simulink model "gm_spec_avg_CRD_vs2"  (R2025b)
settings: Solver=FixedStepDiscrete  StartTime=0.0  StopTime=0.0005  FixedStep=1.66666666666667e-08  RelTol=1e-3
undefined symbols (not defined in the file or in its folder): chirp_counts, chirp_outputs, clk, clk_enable, FFT_LENGTH, Fs, h, reset, specAvg
libraries: simulink x30, hdlmdlgenlib x4, dsphdlsigops2 x2, dsphdlxfrm2 x1, hdlsllib x1, vivadosimlib x1
(part 1 of 2)
settings Model: FPTRunName=BaselineRun  Creator=caleb  LastModifiedBy=caleb
settings OptimizationCC: BlockReduction=off  ConditionallyExecuteInputs=off  DefaultParameterBehavior=Inlined  OptimizeBlockIOStorage=off  EnhancedBackFolding=on  PassReuseOutputArgsThreshold=0.0  OptimizeBlockOrder=speed  DifferentSizesBufferReuse=on
settings DebuggingCC: SignalRangeChecking=warning  AlgebraicLoopMsg=error  InheritedTsInSrcMsg=none  SingleTaskRateTransMsg=error  ParameterTunabilityLossMsg=error
settings HardwareCC: ProdBitPerPointer=32.0  ProdBitPerSizeT=32.0  ProdBitPerPtrDiffT=32.0  ProdLargestAtomicFloat=None  ProdIntDivRoundTo=Undefined  ProdEndianess=Unspecified  ProdWordSize=32.0  ProdHWDeviceType=ASIC/FPGA->ASIC/FPGA  TargetBitPerPointer=64.0  TargetBitPerSizeT=64.0  TargetBitPerPtrDiffT=64.0  TargetLongLongMode=on  TargetIntDivRoundTo=Zero  TargetEndianess=LittleEndian  TargetWordSize=64.0  TargetHWDeviceType=Generic->Custom  ProdEqTarget=off
settings SFSimCC: MATLABDynamicMemAlloc=off
settings RTWCC: GPUComputeCapability=3.5
settings CodeAppCC: ForceParamTrailComments=on  MaxIdLength=256.0  OperatorAnnotations=on

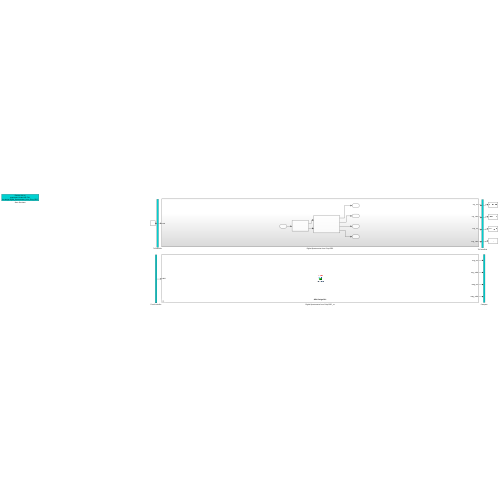
[thumbnail: Simulink's stored preview of the top-level diagram]
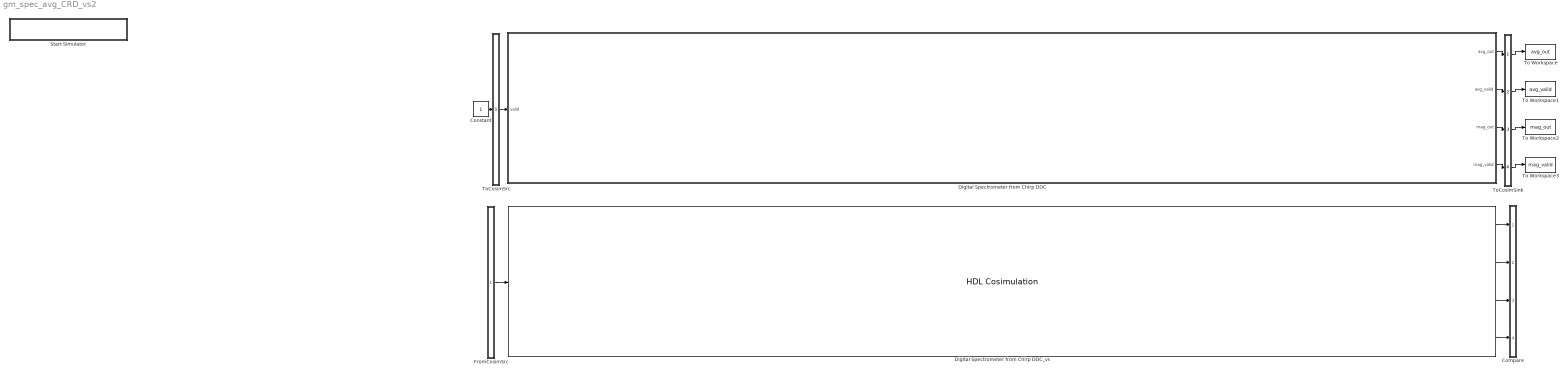
== system gm_spec_avg_CRD_vs2 ==
  Compare : Subsystem
      mask Display: disp('')
  Constant : Constant  OutDataTypeStr=boolean  SampleTime=1/Fs
  Digital Spectrometer from Chirp DDC : Subsystem
  Digital Spectrometer from Chirp DDC_vs : vivadosimlib/HDL Cosimulation  PortPaths=/Digital_Spectrometer_from_Chirp_DDC/valid;/Digital_Spectrometer_from_Chirp_DDC/avg_out;/Digital_Spectrometer_from_Chirp_DDC/avg_valid;/Digital_Spectrometer_from_Chirp_DDC/mag_out;/Digital_Spectrometer_from_Chirp_DDC/mag_valid  PortModes=[1 2 2 2 2 ]  PortTimes=[-1 3.333333333333333403075202767094908917755446964292787015438079834e-08 3.333333333333333403075202767094908917755446964292787015438079834e-08 3.333333333333333403075202767094908917755446964292787015438079834e-08 3.333333333333333403075202767094908917755446964292787015438079834e-08 ]  PortSigns=[-1 1 0 1 0 ]  PortFracLengths=[0,4,0,15,0]  PortWordLengths=[-1,32,1,26,1]  PortHDLWordSizes=[1,32,1,26,1]  CommLocal=on  CommSharedMemory=on  CommPortNumber=4449  CommShowInfo=on  ClockPaths=clk;clk_enable;reset;  ClockModes=[2 4 3]  ClockTimes=[1e-08 3.7e-08 2.7e-08]  TclPostSimCommand="puts \"done\""  TimingMode=ns  TimingScaleFactor=600000000  idxCellArray={'UNUSED_VAR'}  CosimBypass=Full Simulation  AllowDirectFeedthrough=on  ProductName=EDA Simulator Link VS  RunAutoTimescale=off  HdlClocks=0  PreRunTime=40  PreRunTimeUnit=ns
  FromCosimSrc : Subsystem
      mask Display: disp('')
  Start Simulator : Subsystem
      settings: OpenFcn=|
      | cosimDirName = pwd;
      | cd 'C:\VHDL\spec_avg\hdlsrc\spec_avg_CRD';
      | [s,r] = system('vivado -mode batch -source gm_spec_avg_CRD_vs.tcl','-echo');
      | cd (cosimDirName);
      | clear cosimDirName;
      | if s
      |    error('Failed to create Vivado HDL design DLL using script gm_spec_avg_CRD_vs.tcl.');
      | end
      mask Display: disp('Double-click to\nregenerate Vivado HDL DLL\nfor design Digital_Spectrometer_from_Chirp_DDC')
  To Workspace : ToWorkspace  VariableName=avg_out  SampleTime=-1
      settings: Save2DSignal=2-D array (concatenate along first dimension)
  To Workspace1 : ToWorkspace  VariableName=avg_valid  SampleTime=-1
      settings: Save2DSignal=2-D array (concatenate along first dimension)
  To Workspace2 : ToWorkspace  VariableName=mag_out  SampleTime=-1
      settings: Save2DSignal=2-D array (concatenate along first dimension)
  To Workspace3 : ToWorkspace  VariableName=mag_valid  SampleTime=-1
      settings: Save2DSignal=2-D array (concatenate along first dimension)
  ToCosimSink : Subsystem
      mask Display: disp('')
  ToCosimSrc : Subsystem
      mask Display: disp('')
  wires:
  ToCosimSrc/1(out1) -> Digital Spectrometer from Chirp DDC/1(valid)
  Digital Spectrometer from Chirp DDC/1(avg_out) -> ToCosimSink/1(in1)
  Digital Spectrometer from Chirp DDC/2(avg_valid) -> ToCosimSink/2(in2)
  Digital Spectrometer from Chirp DDC/3(mag_out) -> ToCosimSink/3(in3)
  Digital Spectrometer from Chirp DDC/4(mag_valid) -> ToCosimSink/4(in4)
  Constant/1 -> ToCosimSrc/1(in1)
  ToCosimSink/1(out1) -> To Workspace/1
  ToCosimSink/2(out2) -> To Workspace1/1
  ToCosimSink/3(out3) -> To Workspace2/1
  ToCosimSink/4(out4) -> To Workspace3/1
  FromCosimSrc/1(out1) -> Digital Spectrometer from Chirp DDC_vs/1
  Digital Spectrometer from Chirp DDC_vs/1 -> Compare/1(in1)
  Digital Spectrometer from Chirp DDC_vs/2 -> Compare/2(in2)
  Digital Spectrometer from Chirp DDC_vs/3 -> Compare/3(in3)
  Digital Spectrometer from Chirp DDC_vs/4 -> Compare/4(in4)

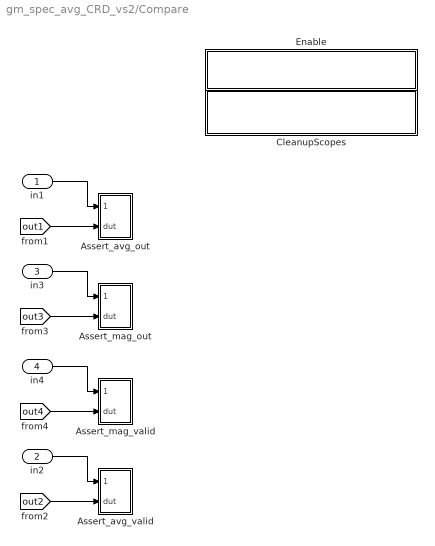
== system gm_spec_avg_CRD_vs2/Compare ==
  in1 : Inport
  in2 : Inport  Port=2
  in3 : Inport  Port=3
  in4 : Inport  Port=4
  Assert_avg_out : Subsystem
  Assert_avg_valid : Subsystem
  Assert_mag_out : Subsystem
  Assert_mag_valid : Subsystem
  CleanupScopes : Subsystem
      settings: OpenFcn=|
      | blkName = gcb; %self block
      | idx = regexp(blkName, '/CleanupScopes$', 'once');
      | blkParent = blkName(1:idx-1);
      | blks=find_system(blkParent, 'LookUnderMasks', 'all','blocktype', 'Scope');
      | for itr = 1:length(blks)
      | 	 hScopeCfg = get_param(blks{itr},'ScopeConfiguration');
      | 	 hScopeCfg.Visible = ~ hScopeCfg.Visible;
      | end
      | drawnow;
      mask Display: fprintf(message('hdlcoder:cosim:vnl_dblclick').getString());
  Enable : Subsystem
      settings: OpenFcn=|
      | blkName = gcb;
      | idx = regexp(blkName, '/Enable$', 'once');
      | blkParent = blkName(1:idx-1);
      | blks=find_system(blkParent, 'LookUnderMasks', 'all','blocktype', 'Assertion');
      | e = get_param(blks{1}, 'Enabled');
      | if strcmp(e, 'on'), f= 'off';, else, f = 'on';, end
      | for ii=1:length(blks), set_param(blks{ii}, 'Enabled', f);, end
      | set_param(gcb, 'MaskDisplay',['fprintf(message(''hdlcoder:cosim:vnl_dblclick_assertions'',','''',upper(e),'''',').getString())']);
      mask Display: fprintf(message('hdlcoder:cosim:vnl_dblclick_assertions','OFF').getString());
  wires:
  in1/1 -> Assert_avg_out/1(cosim)
  [out4] -> Assert_mag_valid/2(dut)
  [out1] -> Assert_avg_out/2(dut)
  in3/1 -> Assert_mag_out/1(cosim)
  [out2] -> Assert_avg_valid/2(dut)
  [out3] -> Assert_mag_out/2(dut)
  in4/1 -> Assert_mag_valid/1(cosim)
  in2/1 -> Assert_avg_valid/1(cosim)

== system gm_spec_avg_CRD_vs2/Digital Spectrometer from Chirp DDC ==
  valid : Inport  OutDataTypeStr=boolean  PortDimensions=1  SampleTime=1.66666666666667e-08
  DDC : Subsystem
  Digital Spectrometer : Subsystem
  avg_out : Outport  SampleTime=3.33333333333333e-08
  avg_valid : Outport  Port=2  SampleTime=3.33333333333333e-08
  mag_out : Outport  Port=3  SampleTime=3.33333333333333e-08
  mag_valid : Outport  Port=4  SampleTime=3.33333333333333e-08
  wires:
  Digital Spectrometer/4(mag_valid) -> mag_valid/1
  Digital Spectrometer/3(mag_out) -> mag_out/1
  Digital Spectrometer/2(avg_valid) -> avg_valid/1
  DDC/2(valid_out) -> Digital Spectrometer/2(valid_in)
  DDC/1(signal_out) -> Digital Spectrometer/1(signal_in)
  valid/1 -> DDC/1(valid)
  Digital Spectrometer/1(avg_out) -> avg_out/1

== system gm_spec_avg_CRD_vs2/FromCosimSrc ==
  out1 : Outport
  wires:
  [in1] -> out1/1

== system gm_spec_avg_CRD_vs2/Start Simulator ==

== system gm_spec_avg_CRD_vs2/ToCosimSink ==
  in1 : Inport
  in2 : Inport  Port=2
  in3 : Inport  Port=3
  in4 : Inport  Port=4
  out1 : Outport
  out2 : Outport  Port=2
  out3 : Outport  Port=3
  out4 : Outport  Port=4
  tag scope: out1=global, out2=global, out3=global, out4=global
  wires:
  in1/1 -> out1/1, [out1]
  in2/1 -> out2/1, [out2]
  in3/1 -> out3/1, [out3]
  in4/1 -> out4/1, [out4]

== system gm_spec_avg_CRD_vs2/ToCosimSrc ==
  in1 : Inport
  out1 : Outport
  tag scope: in1=global
  wires:
  in1/1 -> out1/1, [in1]

== system gm_spec_avg_CRD_vs2/Compare/Assert_avg_out ==
  cosim : Inport
  dut : Inport  Port=2
  AssertEq : Assertion
  Compare To Zero : simulink/Logic and Bit Operations/Compare To Zero  relop===  OutDataTypeStr=boolean
  Relational Operator : RelationalOperator  Operator===  OutDataTypeStr=boolean  InputSameDT=off
  compare: avg_out : Scope  NumInputPorts=3
      settings: ActiveDisplayYMinimum=-29.585937499999993  ActiveDisplayYMaximum=229.3984375
  wires:
  Compare To Zero/1 -> compare: avg_out/3  "err"
  Relational Operator/1 -> Compare To Zero/1, AssertEq/1
  cosim/1 -> compare: avg_out/1, Relational Operator/1  "cosim"
  dut/1 -> compare: avg_out/2, Relational Operator/2  "dut ref"

== system gm_spec_avg_CRD_vs2/Compare/Assert_avg_valid ==
  cosim : Inport
  dut : Inport  Port=2
  AssertEq : Assertion
  Compare To Zero : simulink/Logic and Bit Operations/Compare To Zero  relop===  OutDataTypeStr=boolean
  Relational Operator : RelationalOperator  Operator===  OutDataTypeStr=boolean  InputSameDT=off
  compare: avg_valid : Scope  NumInputPorts=3
      settings: ActiveDisplayYMinimum=-5  ActiveDisplayYMaximum=5
  wires:
  Compare To Zero/1 -> compare: avg_valid/3  "err"
  Relational Operator/1 -> Compare To Zero/1, AssertEq/1
  cosim/1 -> compare: avg_valid/1, Relational Operator/1  "cosim"
  dut/1 -> compare: avg_valid/2, Relational Operator/2  "dut ref"

== system gm_spec_avg_CRD_vs2/Compare/Assert_mag_out ==
  cosim : Inport
  dut : Inport  Port=2
  AssertEq : Assertion
  Compare To Zero : simulink/Logic and Bit Operations/Compare To Zero  relop===  OutDataTypeStr=boolean
  Relational Operator : RelationalOperator  Operator===  OutDataTypeStr=boolean  InputSameDT=off
  compare: mag_out : Scope  NumInputPorts=3
      settings: ActiveDisplayYMinimum=-5  ActiveDisplayYMaximum=5
  wires:
  Compare To Zero/1 -> compare: mag_out/3  "err"
  Relational Operator/1 -> Compare To Zero/1, AssertEq/1
  cosim/1 -> compare: mag_out/1, Relational Operator/1  "cosim"
  dut/1 -> compare: mag_out/2, Relational Operator/2  "dut ref"

== system gm_spec_avg_CRD_vs2/Compare/Assert_mag_valid ==
  cosim : Inport
  dut : Inport  Port=2
  AssertEq : Assertion
  Compare To Zero : simulink/Logic and Bit Operations/Compare To Zero  relop===  OutDataTypeStr=boolean
  Relational Operator : RelationalOperator  Operator===  OutDataTypeStr=boolean  InputSameDT=off
  compare: mag_valid : Scope  NumInputPorts=3
      settings: ActiveDisplayYMinimum=-5  ActiveDisplayYMaximum=5
  wires:
  Compare To Zero/1 -> compare: mag_valid/3  "err"
  Relational Operator/1 -> Compare To Zero/1, AssertEq/1
  cosim/1 -> compare: mag_valid/1, Relational Operator/1  "cosim"
  dut/1 -> compare: mag_valid/2, Relational Operator/2  "dut ref"

== system gm_spec_avg_CRD_vs2/Compare/CleanupScopes ==

== system gm_spec_avg_CRD_vs2/Compare/Enable ==

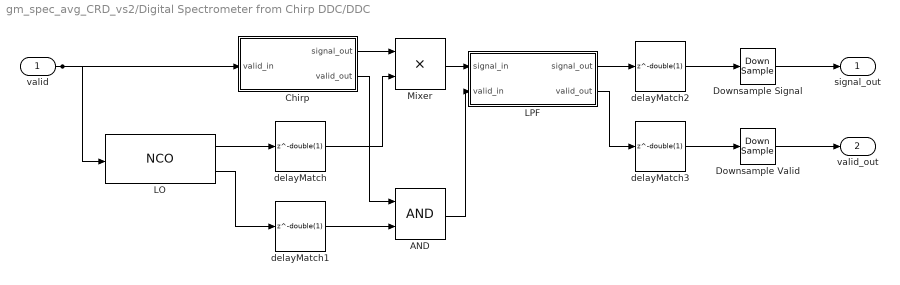
== system gm_spec_avg_CRD_vs2/Digital Spectrometer from Chirp DDC/DDC ==
  valid : Inport  OutDataTypeStr=boolean  PortDimensions=1  SampleTime=1.66666666666667e-08
  AND : Logic  AllPortsSameDT=off  OutDataTypeStr=boolean  SampleTime=1.66666666666667e-08
  Chirp : Subsystem
  Downsample Signal : DownSample  N=double(2)  phase=double(0)  RateOptions=Allow multirate processing  AllowArbitraryFixedInput=on
  Downsample Valid : DownSample  N=double(2)  phase=double(0)  RateOptions=Allow multirate processing  AllowArbitraryFixedInput=on
  LO : dsphdlsigops2/NCO  PhaseIncrementSource=Property  PhaseIncrement=phIncr  PhaseOffsetSource=Property  PhaseOffset=phOff  DitherSource=Property  NumDitherBits=ditherBits  SamplesPerFrame=1  LUTCompress=off  ResetAction=off  Waveform=Cosine  PhasePort=off  SimulateUsing=Code generation  AccumulatorWL=N  PhaseQuantization=on  NumQuantizerAccumulatorBits=Q  OutputDataType=Binary point scaling  OutputWL=16  OutputFL=14
  LPF : Subsystem
  Mixer : Product  Inputs=**  OutDataTypeStr=fixdt(1, 16, 14)  SampleTime=1.66666666666667e-08
  delayMatch{,1..3} (4 alike) : Delay  DelayLength=double(1)  InitialCondition=0  SampleTime=1.66666666666667e-08
  signal_out : Outport  SampleTime=3.33333333333333e-08  VectorParamsAs1DForOutWhenUnconnected=off
  valid_out : Outport  Port=2  SampleTime=3.33333333333333e-08  VectorParamsAs1DForOutWhenUnconnected=off
  wires:
  Downsample Valid/1 -> valid_out/1
  Downsample Signal/1 -> signal_out/1
  delayMatch3/1 -> Downsample Valid/1
  delayMatch2/1 -> Downsample Signal/1
  LPF/2(valid_out) -> delayMatch3/1
  LPF/1(signal_out) -> delayMatch2/1
  AND/1 -> LPF/2(valid_in)
  Mixer/1 -> LPF/1(signal_in)
  delayMatch1/1 -> AND/2
  Chirp/2(valid_out) -> AND/1
  Chirp/1(signal_out) -> Mixer/1
  LO/2 -> delayMatch1/1
  LO/1 -> delayMatch/1
  delayMatch/1 -> Mixer/2
  valid/1 -> LO/1, Chirp/1(valid_in)

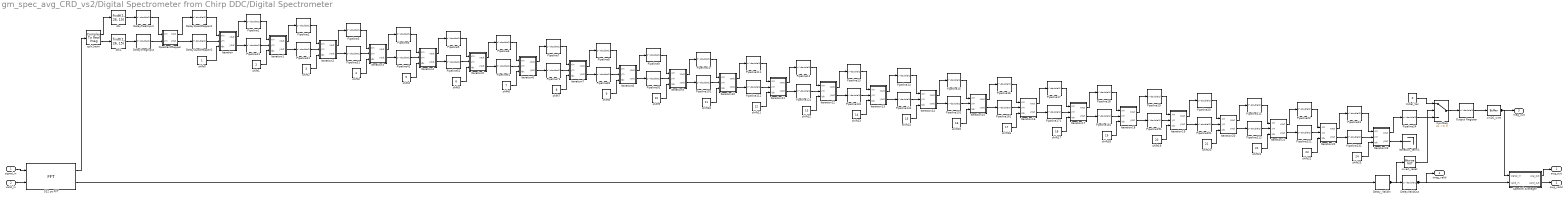
== system gm_spec_avg_CRD_vs2/Digital Spectrometer from Chirp DDC/Digital Spectrometer ==
  signal_in : Inport  OutDataTypeStr=fixdt(1, 16, 15)  PortDimensions=1  SampleTime=3.33333333333333e-08
  valid_in : Inport  Port=2  OutDataTypeStr=boolean  PortDimensions=1  SampleTime=3.33333333333333e-08
  512 pt FFT : dsphdlxfrm2/FFT  Architecture=Streaming Radix 2^2  FFTLengthSource=Property  FFTLength=FFT_LENGTH  FFTLengthMax=1024  ComplexMultiplication=Use 4 multipliers and 2 adders  BitReversedOutput=off  BitReversedInput=off  Normalize=off  SimulateUsing=Code generation  RoundingMethod=Floor  ResetInputPort=off  StartOutputPort=off  EndOutputPort=off
  DelayImagInput : Delay  DelayLength=double(1)  InitialCondition=0  SampleTime=3.33333333333333e-08
  DelayQuadMapper1 : Delay  DelayLength=double(1)  InitialCondition=0  SampleTime=3.33333333333333e-08
  DelayQuadMapper2 : Delay  DelayLength=double(1)  InitialCondition=0  SampleTime=3.33333333333333e-08
  DelayRealInput : Delay  DelayLength=double(1)  InitialCondition=0  SampleTime=3.33333333333333e-08
  DelayValidOut : Delay  DelayLength=double(1)  InitialCondition=0  SampleTime=3.33333333333333e-08
  Delay_ValidIn : Delay  DelayLength=double(27)  InitialCondition=0  SampleTime=3.33333333333333e-08
  Initial_Val : Constant  Value=0  OutDataTypeStr=fixdt(1, 26, 15)  SampleTime=3.33333333333333e-08
  Iteration : Subsystem
  Iteration1 : Subsystem
  Iteration10 : Subsystem
  Iteration11 : Subsystem
  Iteration12 : Subsystem
  Iteration13 : Subsystem
  Iteration14 : Subsystem
  Iteration15 : Subsystem
  Iteration16 : Subsystem
  Iteration17 : Subsystem
  Iteration18 : Subsystem
  Iteration19 : Subsystem
  Iteration2 : Subsystem
  Iteration20 : Subsystem
  Iteration21 : Subsystem
  Iteration22 : Subsystem
  Iteration23 : Subsystem
  Iteration3 : Subsystem
  Iteration4 : Subsystem
  Iteration5 : Subsystem
  Iteration6 : Subsystem
  Iteration7 : Subsystem
  Iteration8 : Subsystem
  Iteration9 : Subsystem
  Iteration_term1 : Terminator
  Output Register : Delay  DelayLength=double(1)  InitialCondition=0  SampleTime=3.33333333333333e-08
  Pipeline{1..24,31,41,51,61,71,81,91,101,111..112,121,131,141,151,161,171,181,191,201,211..212,221,231} (47 alike) : Delay  DelayLength=double(1)  InitialCondition=0  SampleTime=3.33333333333333e-08
  QuadrantMapper : Subsystem
  Spectral Averager : Subsystem
  cplx2reim : ComplexToRealImag  SampleTime=3.33333333333333e-08
  dtc : DataTypeConversion  OutDataTypeStr=fixdt(1, 26, 15)  SampleTime=3.33333333333333e-08  SaturateOnIntegerOverflow=off  RndMeth=Floor
  dtc1 : DataTypeConversion  OutDataTypeStr=fixdt(1, 26, 15)  SampleTime=3.33333333333333e-08  SaturateOnIntegerOverflow=off  RndMeth=Floor
  invert_reset : simulink/Logic and Bit Operations/Bitwise Operator  logicop=NOT  UseBitMask=off  BitMask=double(0)  BitMaskRealWorld=Real World Value
  muxMag : Switch  Criteria=u2 ~= 0  Threshold="fi(0,0,1,0,\"hex\",\"0\")"  OutDataTypeStr=fixdt(1, 26, 15)  SampleTime=3.33333333333333e-08  SaturateOnIntegerOverflow=off  InputSameDT=off
  shift0 : Constant  VectorParams1D=off  OutDataTypeStr=fixdt(0, 6, 0)  SampleTime=3.33333333333333e-08
  shift1 : Constant  Value=2  VectorParams1D=off  OutDataTypeStr=fixdt(0, 6, 0)  SampleTime=3.33333333333333e-08
  shift10 : Constant  Value=11  VectorParams1D=off  OutDataTypeStr=fixdt(0, 6, 0)  SampleTime=3.33333333333333e-08
  shift11 : Constant  Value=12  VectorParams1D=off  OutDataTypeStr=fixdt(0, 6, 0)  SampleTime=3.33333333333333e-08
  shift12 : Constant  Value=13  VectorParams1D=off  OutDataTypeStr=fixdt(0, 6, 0)  SampleTime=3.33333333333333e-08
  shift13 : Constant  Value=14  VectorParams1D=off  OutDataTypeStr=fixdt(0, 6, 0)  SampleTime=3.33333333333333e-08
  shift14 : Constant  Value=15  VectorParams1D=off  OutDataTypeStr=fixdt(0, 6, 0)  SampleTime=3.33333333333333e-08
  shift15 : Constant  Value=16  VectorParams1D=off  OutDataTypeStr=fixdt(0, 6, 0)  SampleTime=3.33333333333333e-08
  shift16 : Constant  Value=17  VectorParams1D=off  OutDataTypeStr=fixdt(0, 6, 0)  SampleTime=3.33333333333333e-08
  shift17 : Constant  Value=18  VectorParams1D=off  OutDataTypeStr=fixdt(0, 6, 0)  SampleTime=3.33333333333333e-08
  shift18 : Constant  Value=19  VectorParams1D=off  OutDataTypeStr=fixdt(0, 6, 0)  SampleTime=3.33333333333333e-08
  shift19 : Constant  Value=20  VectorParams1D=off  OutDataTypeStr=fixdt(0, 6, 0)  SampleTime=3.33333333333333e-08
  shift2 : Constant  Value=3  VectorParams1D=off  OutDataTypeStr=fixdt(0, 6, 0)  SampleTime=3.33333333333333e-08
  shift20 : Constant  Value=21  VectorParams1D=off  OutDataTypeStr=fixdt(0, 6, 0)  SampleTime=3.33333333333333e-08
  shift21 : Constant  Value=22  VectorParams1D=off  OutDataTypeStr=fixdt(0, 6, 0)  SampleTime=3.33333333333333e-08
  shift22 : Constant  Value=23  VectorParams1D=off  OutDataTypeStr=fixdt(0, 6, 0)  SampleTime=3.33333333333333e-08
  shift23 : Constant  Value=24  VectorParams1D=off  OutDataTypeStr=fixdt(0, 6, 0)  SampleTime=3.33333333333333e-08
  shift3 : Constant  Value=4  VectorParams1D=off  OutDataTypeStr=fixdt(0, 6, 0)  SampleTime=3.33333333333333e-08
  shift4 : Constant  Value=5  VectorParams1D=off  OutDataTypeStr=fixdt(0, 6, 0)  SampleTime=3.33333333333333e-08
  shift5 : Constant  Value=6  VectorParams1D=off  OutDataTypeStr=fixdt(0, 6, 0)  SampleTime=3.33333333333333e-08
  shift6 : Constant  Value=7  VectorParams1D=off  OutDataTypeStr=fixdt(0, 6, 0)  SampleTime=3.33333333333333e-08
  shift7 : Constant  Value=8  VectorParams1D=off  OutDataTypeStr=fixdt(0, 6, 0)  SampleTime=3.33333333333333e-08
  shift8 : Constant  Value=9  VectorParams1D=off  OutDataTypeStr=fixdt(0, 6, 0)  SampleTime=3.33333333333333e-08
  shift9 : Constant  Value=10  VectorParams1D=off  OutDataTypeStr=fixdt(0, 6, 0)  SampleTime=3.33333333333333e-08
  xin26_wire : hdlmdlgenlib/Buffer
  avg_out : Outport  SampleTime=3.33333333333333e-08
  avg_valid : Outport  Port=2  SampleTime=3.33333333333333e-08
  mag_out : Outport  Port=3  SampleTime=3.33333333333333e-08
  mag_valid : Outport  Port=4  SampleTime=3.33333333333333e-08
  wires:
  Spectral Averager/2(valid_out) -> avg_valid/1
  Spectral Averager/1(avg_out) -> avg_out/1
  xin26_wire/1 -> mag_out/1, Spectral Averager/1(signal_in)
  Output Register/1 -> xin26_wire/1
  muxMag/1 -> Output Register/1
  DelayValidOut/1 -> mag_valid/1, Spectral Averager/2(valid_in)
  Pipeline24/1 -> muxMag/3
  Initial_Val/1 -> muxMag/1
  Delay_ValidIn/1 -> DelayValidOut/1, invert_reset/1
  Iteration23/2(yout) -> Iteration_term1/1
  Iteration23/1(xout) -> Pipeline24/1
  shift23/1 -> Iteration23/3(idx)
  Pipeline231/1 -> Iteration23/2(yin)
  Pipeline23/1 -> Iteration23/1(xin)
  Iteration22/2(yout) -> Pipeline231/1
  Iteration22/1(xout) -> Pipeline23/1
  shift22/1 -> Iteration22/3(idx)
  Pipeline221/1 -> Iteration22/2(yin)
  Pipeline22/1 -> Iteration22/1(xin)
  Iteration21/2(yout) -> Pipeline221/1
  Iteration21/1(xout) -> Pipeline22/1
  shift21/1 -> Iteration21/3(idx)
  Pipeline211/1 -> Iteration21/1(xin)
  Iteration20/2(yout) -> Pipeline212/1
  Iteration20/1(xout) -> Pipeline211/1
  shift20/1 -> Iteration20/3(idx)
  Pipeline20/1 -> Iteration20/1(xin)
  Iteration19/1(xout) -> Pipeline20/1
  shift19/1 -> Iteration19/3(idx)
  Pipeline191/1 -> Iteration19/2(yin)
  Pipeline19/1 -> Iteration19/1(xin)
  Iteration18/1(xout) -> Pipeline19/1
  shift18/1 -> Iteration18/3(idx)
  Pipeline212/1 -> Iteration21/2(yin)
  Pipeline181/1 -> Iteration18/2(yin)
  Pipeline18/1 -> Iteration18/1(xin)
  Iteration17/2(yout) -> Pipeline181/1
  Pipeline17/1 -> Iteration17/1(xin)
  Iteration16/2(yout) -> Pipeline171/1
  Iteration16/1(xout) -> Pipeline17/1
  shift16/1 -> Iteration16/3(idx)
  Pipeline161/1 -> Iteration16/2(yin)
  Pipeline16/1 -> Iteration16/1(xin)
  Iteration15/2(yout) -> Pipeline161/1
  Iteration15/1(xout) -> Pipeline16/1
  shift15/1 -> Iteration15/3(idx)
  Pipeline151/1 -> Iteration15/2(yin)
  Pipeline15/1 -> Iteration15/1(xin)
  Iteration14/2(yout) -> Pipeline151/1
  Iteration14/1(xout) -> Pipeline15/1
  shift14/1 -> Iteration14/3(idx)
  Pipeline141/1 -> Iteration14/2(yin)
  Pipeline14/1 -> Iteration14/1(xin)
  Iteration13/2(yout) -> Pipeline141/1
  shift13/1 -> Iteration13/3(idx)
  Pipeline131/1 -> Iteration13/2(yin)
  Pipeline13/1 -> Iteration13/1(xin)
  Iteration12/2(yout) -> Pipeline131/1
  Iteration12/1(xout) -> Pipeline13/1
  shift12/1 -> Iteration12/3(idx)
  Pipeline12/1 -> Iteration12/1(xin)
  Iteration11/1(xout) -> Pipeline12/1
  shift11/1 -> Iteration11/3(idx)
  Pipeline112/1 -> Iteration11/2(yin)
  Iteration10/2(yout) -> Pipeline112/1
  Iteration10/1(xout) -> Pipeline111/1
  shift10/1 -> Iteration10/3(idx)
  Iteration9/1(xout) -> Pipeline10/1
  Pipeline9/1 -> Iteration9/1(xin)
  Iteration8/2(yout) -> Pipeline91/1
  Pipeline8/1 -> Iteration8/1(xin)
  shift7/1 -> Iteration7/3(idx)
  Pipeline7/1 -> Iteration7/1(xin)
  Pipeline6/1 -> Iteration6/1(xin)
  Iteration7/2(yout) -> Pipeline81/1
  Pipeline101/1 -> Iteration10/2(yin)
  Iteration5/1(xout) -> Pipeline6/1
  shift5/1 -> Iteration5/3(idx)
  Pipeline91/1 -> Iteration9/2(yin)
  Pipeline5/1 -> Iteration5/1(xin)
  shift6/1 -> Iteration6/3(idx)
  Iteration11/2(yout) -> Pipeline121/1
  Pipeline201/1 -> Iteration20/2(yin)
  Iteration6/2(yout) -> Pipeline71/1
  Pipeline41/1 -> Iteration4/2(yin)
  Pipeline4/1 -> Iteration4/1(xin)
  Pipeline171/1 -> Iteration17/2(yin)
  Iteration3/2(yout) -> Pipeline41/1
  invert_reset/1 -> muxMag/2
  Iteration3/1(xout) -> Pipeline4/1
  Pipeline61/1 -> Iteration6/2(yin)
  shift8/1 -> Iteration8/3(idx)
  shift3/1 -> Iteration3/3(idx)
  Pipeline31/1 -> Iteration3/2(yin)
  Iteration18/2(yout) -> Pipeline191/1
  Pipeline3/1 -> Iteration3/1(xin)
  shift4/1 -> Iteration4/3(idx)
  Pipeline71/1 -> Iteration7/2(yin)
  Iteration2/2(yout) -> Pipeline31/1
  Iteration2/1(xout) -> Pipeline3/1
  shift2/1 -> Iteration2/3(idx)
  Pipeline111/1 -> Iteration11/1(xin)
  Pipeline51/1 -> Iteration5/2(yin)
  Iteration1/2(yout) -> Pipeline21/1
  Iteration6/1(xout) -> Pipeline7/1
  Iteration1/1(xout) -> Pipeline2/1
  shift1/1 -> Iteration1/3(idx)
  Iteration17/1(xout) -> Pipeline18/1
  Pipeline10/1 -> Iteration10/1(xin)
  Pipeline11/1 -> Iteration1/2(yin)
  Pipeline1/1 -> Iteration1/1(xin)
  Pipeline21/1 -> Iteration2/2(yin)
  Iteration7/1(xout) -> Pipeline8/1
  Iteration8/1(xout) -> Pipeline9/1
  Iteration/2(yout) -> Pipeline11/1
  Pipeline121/1 -> Iteration12/2(yin)
  Pipeline2/1 -> Iteration2/1(xin)
  Iteration19/2(yout) -> Pipeline201/1
  shift9/1 -> Iteration9/3(idx)
  shift0/1 -> Iteration/3(idx)
  Iteration5/2(yout) -> Pipeline61/1
  DelayQuadMapper2/1 -> Iteration/2(yin)
  Pipeline81/1 -> Iteration8/2(yin)
  DelayQuadMapper1/1 -> Iteration/1(xin)
  Iteration13/1(xout) -> Pipeline14/1
  QuadrantMapper/1(xout) -> DelayQuadMapper1/1
  DelayImagInput/1 -> QuadrantMapper/2(yin)
  DelayRealInput/1 -> QuadrantMapper/1(xin)
  shift17/1 -> Iteration17/3(idx)
  QuadrantMapper/2(yout) -> DelayQuadMapper2/1
  Iteration9/2(yout) -> Pipeline101/1
  dtc1/1 -> DelayImagInput/1
  Iteration4/1(xout) -> Pipeline5/1
  dtc/1 -> DelayRealInput/1
  cplx2reim/1 -> dtc/1
  Iteration4/2(yout) -> Pipeline51/1
  Iteration/1(xout) -> Pipeline1/1
  valid_in/1 -> 512 pt FFT/2
  512 pt FFT/1 -> cplx2reim/1
  512 pt FFT/2 -> Delay_ValidIn/1
  cplx2reim/2 -> dtc1/1
  signal_in/1 -> 512 pt FFT/1

== system gm_spec_avg_CRD_vs2/Digital Spectrometer from Chirp DDC/DDC/Chirp ==
  valid_in : Inport  OutDataTypeStr=boolean  PortDimensions=1  SampleTime=1.66666666666667e-08
  1-D Lookup Table1 : Subsystem
  Constant : Constant  Value=35.791015625  OutDataTypeStr=fixdt(0, 16, 10)  SampleTime=1.66666666666667e-08
  Counter Limited : Subsystem  mask(Counter Limited){uplimit=double(30000), tsamp=double(1.6666666666666667e-08)}
      mask prompts: uplimit "Simulink:masks:UpperLimit_MP"; tsamp "Simulink:masks:SampleTime_MP"
      mask help: Simulink:masks:CounterLimited_MD
      mask init:
      | nbits = double(16);
      | tsamp = double(1.6666666666666667e-08);
      | uplimit = double(30000);
  NCO1 : dsphdlsigops2/NCO  PhaseIncrementSource=Input port  PhaseIncrement=phIncr  PhaseOffsetSource=Property  PhaseOffset=phOff  DitherSource=Property  NumDitherBits=ditherBits  SamplesPerFrame=1  LUTCompress=off  ResetAction=off  Waveform=Cosine  PhasePort=off  SimulateUsing=Code generation  AccumulatorWL=N  PhaseQuantization=on  NumQuantizerAccumulatorBits=Q  OutputDataType=Binary point scaling  OutputWL=16  OutputFL=14
  Product : Product  Inputs=**  OutDataTypeStr=uint32  SampleTime=1.66666666666667e-08
  delayMatch : Delay  DelayLength=double(1)  InitialCondition=0  SampleTime=1.66666666666667e-08
  signal_out : Outport  SampleTime=1.66666666666667e-08
  valid_out : Outport  Port=2  SampleTime=1.66666666666667e-08
  wires:
  NCO1/2 -> valid_out/1
  delayMatch/1 -> NCO1/2
  Product/1 -> NCO1/1
  valid_in/1 -> delayMatch/1
  1-D Lookup Table1/1(Out1) -> Product/2
  Counter Limited/1(y) -> 1-D Lookup Table1/1(In1)
  Constant/1 -> Product/1
  NCO1/1 -> signal_out/1

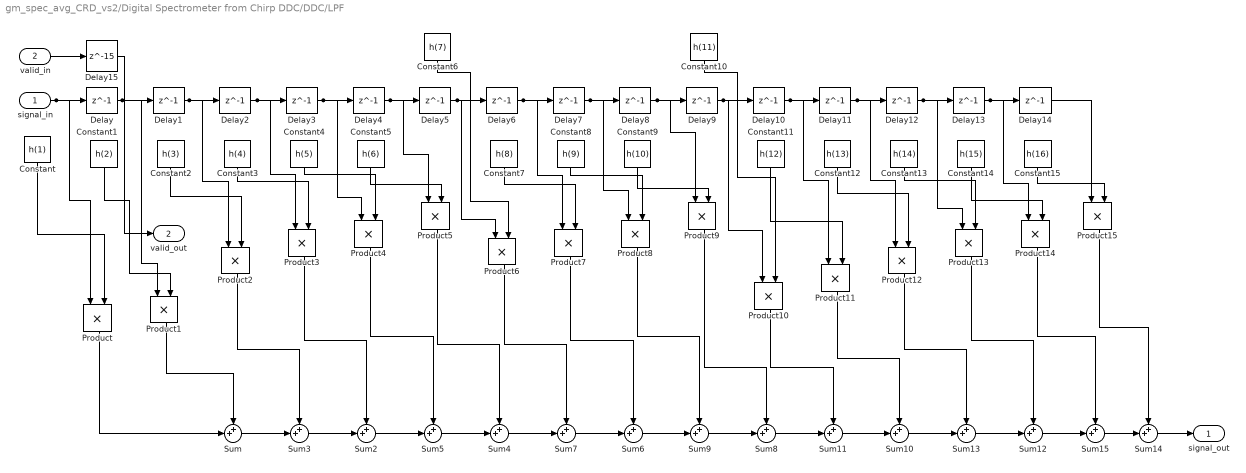
== system gm_spec_avg_CRD_vs2/Digital Spectrometer from Chirp DDC/DDC/LPF ==
  signal_in : Inport  OutDataTypeStr=fixdt(1, 16, 14)  PortDimensions=1  SampleTime=1.66666666666667e-08
  valid_in : Inport  Port=2  OutDataTypeStr=boolean  PortDimensions=1  SampleTime=1.66666666666667e-08
  Constant : Constant  Value=h(1)  OutDataTypeStr=fixdt(1,16,4)  SampleTime=1/Fs
  Constant1 : Constant  Value=h(2)  OutDataTypeStr=fixdt(1,16,25)  SampleTime=1/Fs
  Constant10 : Constant  Value=h(11)  OutDataTypeStr=fixdt(0,16,19)  SampleTime=1/Fs
  Constant11 : Constant  Value=h(12)  OutDataTypeStr=fixdt(0,16,23)  SampleTime=1/Fs
  Constant12 : Constant  Value=h(13)  OutDataTypeStr=fixdt(1,16,21)  SampleTime=1/Fs
  Constant13 : Constant  Value=h(14)  OutDataTypeStr=fixdt(1,16,22)  SampleTime=1/Fs
  Constant14 : Constant  Value=h(15)  OutDataTypeStr=fixdt(1,16,25)  SampleTime=1/Fs
  Constant15 : Constant  Value=h(16)  OutDataTypeStr=fixdt(1,16,4)  SampleTime=1/Fs
  Constant2 : Constant  Value=h(3)  OutDataTypeStr=fixdt(1,16,22)  SampleTime=1/Fs
  Constant3 : Constant  Value=h(4)  OutDataTypeStr=fixdt(1,16,21)  SampleTime=1/Fs
  Constant4 : Constant  Value=h(5)  OutDataTypeStr=fixdt(0,16,23)  SampleTime=1/Fs
  Constant5 : Constant  Value=h(6)  OutDataTypeStr=fixdt(0,16,19)  SampleTime=1/Fs
  Constant6 : Constant  Value=h(7)  OutDataTypeStr=fixdt(0,16,18)  SampleTime=1/Fs
  Constant7 : Constant  Value=h(8)  OutDataTypeStr=fixdt(0,16,17)  SampleTime=1/Fs
  Constant8 : Constant  Value=h(9)  OutDataTypeStr=fixdt(0,16,17)  SampleTime=1/Fs
  Constant9 : Constant  Value=h(10)  OutDataTypeStr=fixdt(0,16,18)  SampleTime=1/Fs
  Delay{,1..14} (15 alike) : Delay  DelayLength=1  InitialCondition=0  UseCircularBuffer=on
  Delay15 : Delay  DelayLength=15
  Product : Product  OutDataTypeStr=fixdt(1,16,4)
  Product1 : Product  OutDataTypeStr=fixdt(1,16,25)
  Product10 : Product  OutDataTypeStr=fixdt(1,16,18)
  Product{2,4,11,13} (4 alike) : Product  OutDataTypeStr=fixdt(1,16,22)
  Product12 : Product  OutDataTypeStr=fixdt(1,16,21)
  Product14 : Product  OutDataTypeStr=fixdt(1,16,25)
  Product15 : Product  OutDataTypeStr=fixdt(1,16,4)
  Product3 : Product  OutDataTypeStr=fixdt(1,16,21)
  Product5 : Product  OutDataTypeStr=fixdt(1,16,18)
  Product6 : Product  OutDataTypeStr=fixdt(1,16,17)
  Product7 : Product  OutDataTypeStr=fixdt(1,16,16)
  Product8 : Product  OutDataTypeStr=fixdt(1,16,16)
  Product9 : Product  OutDataTypeStr=fixdt(1,16,17)
  Sum : Sum  Inputs=++|  OutDataTypeStr=fixdt(1,16,25)
  Sum{8,10..15} (7 alike) : Sum  Inputs=++|  OutDataTypeStr=fixdt(1,16,15)
  Sum2 : Sum  Inputs=++|  OutDataTypeStr=fixdt(1,16,21)
  Sum3 : Sum  Inputs=++|  OutDataTypeStr=fixdt(1,16,22)
  Sum4 : Sum  Inputs=++|  OutDataTypeStr=fixdt(1,16,18)
  Sum5 : Sum  Inputs=++|  OutDataTypeStr=fixdt(1,16,21)
  Sum6 : Sum  Inputs=++|  OutDataTypeStr=fixdt(1,16,16)
  Sum7 : Sum  Inputs=++|  OutDataTypeStr=fixdt(1,16,17)
  Sum9 : Sum  Inputs=++|  OutDataTypeStr=fixdt(1,16,16)
  signal_out : Outport  SampleTime=1.66666666666667e-08
  valid_out : Outport  Port=2  SampleTime=1.66666666666667e-08  VectorParamsAs1DForOutWhenUnconnected=off
  wires:
  Sum14/1 -> signal_out/1
  Product15/1 -> Sum14/1
  Delay14/1 -> Product15/1
  Product14/1 -> Sum15/1
  Delay13/1 -> Delay14/1, Product14/1
  Product13/1 -> Sum12/1
  Constant14/1 -> Product14/2
  Product12/1 -> Sum13/1
  Delay11/1 -> Delay12/1, Product12/1
  Sum15/1 -> Sum14/2
  Product11/1 -> Sum10/1
  Constant12/1 -> Product12/2
  Delay10/1 -> Delay11/1, Product11/1
  Product10/1 -> Sum11/1
  Sum9/1 -> Sum8/2
  Delay9/1 -> Delay10/1, Product10/1
  Product9/1 -> Sum8/1
  Constant15/1 -> Product15/2
  Constant10/1 -> Product10/2
  Sum6/1 -> Sum9/2
  Delay8/1 -> Product9/1, Delay9/1
  Product8/1 -> Sum9/1
  Constant13/1 -> Product13/2
  Constant9/1 -> Product9/2
  Sum12/1 -> Sum15/2
  Delay7/1 -> Delay8/1, Product8/1
  Product7/1 -> Sum6/1
  Constant11/1 -> Product11/2
  Constant8/1 -> Product8/2
  Delay6/1 -> Delay7/1, Product7/1
  Sum8/1 -> Sum11/2
  Constant7/1 -> Product7/2
  Sum11/1 -> Sum10/2
  Delay5/1 -> Delay6/1, Product6/1
  Sum7/1 -> Sum6/2
  Product5/1 -> Sum4/1
  Sum2/1 -> Sum5/2
  Delay12/1 -> Delay13/1, Product13/1
  Delay4/1 -> Delay5/1, Product5/1
  Product4/1 -> Sum5/1
  Constant5/1 -> Product5/2
  Sum10/1 -> Sum13/2
  Sum3/1 -> Sum2/2
  Delay3/1 -> Delay4/1, Product4/1
  Product3/1 -> Sum2/1
  Delay2/1 -> Delay3/1, Product3/1
  Sum5/1 -> Sum4/2
  Product2/1 -> Sum3/1
  Constant3/1 -> Product3/2
  Sum/1 -> Sum3/2
  Delay1/1 -> Delay2/1, Product2/1
  Product1/1 -> Sum/1
  Delay15/1 -> valid_out/1
  Sum4/1 -> Sum7/2
  Constant1/1 -> Product1/2
  Product6/1 -> Sum7/1
  Product/1 -> Sum/2
  Delay/1 -> Delay1/1, Product1/1
  Sum13/1 -> Sum12/2
  signal_in/1 -> Delay/1, Product/1
  Constant4/1 -> Product4/2
  valid_in/1 -> Delay15/1
  Constant6/1 -> Product6/2
  Constant/1 -> Product/2
  Constant2/1 -> Product2/2

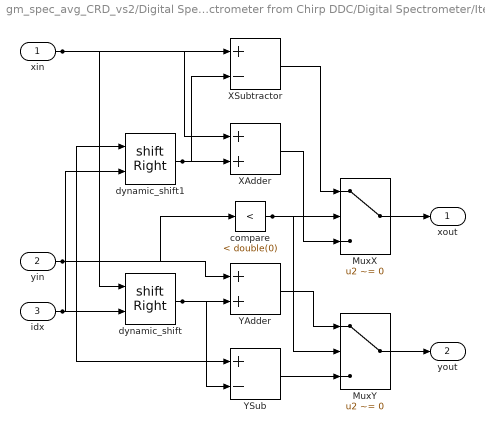
== system gm_spec_avg_CRD_vs2/Digital Spectrometer from Chirp DDC/Digital Spectrometer/Iteration ==
  xin : Inport  OutDataTypeStr=fixdt(1, 26, 15)  SampleTime=3.33333333333333e-08
  yin : Inport  Port=2  OutDataTypeStr=fixdt(1, 26, 15)  SampleTime=3.33333333333333e-08
  idx : Inport  Port=3  OutDataTypeStr=fixdt(0, 6, 0)  SampleTime=3.33333333333333e-08
  MuxX : Switch  Criteria=u2 ~= 0  Threshold="fi(0,0,1,0,\"hex\",\"0\")"  OutDataTypeStr=fixdt(1, 26, 15)  SampleTime=3.33333333333333e-08  SaturateOnIntegerOverflow=off  InputSameDT=off
  MuxY : Switch  Criteria=u2 ~= 0  Threshold="fi(0,0,1,0,\"hex\",\"0\")"  OutDataTypeStr=fixdt(1, 26, 15)  SampleTime=3.33333333333333e-08  SaturateOnIntegerOverflow=off  InputSameDT=off
  XAdder : Sum  OutDataTypeStr=fixdt(1, 26, 15)  SampleTime=3.33333333333333e-08
  XSubtractor : Sum  Inputs=+-  OutDataTypeStr=fixdt(1, 26, 15)  AccumDataTypeStr=fixdt(1, 26, 15)  SampleTime=3.33333333333333e-08
  YAdder : Sum  OutDataTypeStr=fixdt(1, 26, 15)  SampleTime=3.33333333333333e-08
  YSub : Sum  Inputs=+-  OutDataTypeStr=fixdt(1, 26, 15)  AccumDataTypeStr=fixdt(1, 26, 15)  SampleTime=3.33333333333333e-08
  compare : simulink/Logic and Bit Operations/Compare To Constant  relop=<  const=double(0)  OutDataTypeStr=boolean
  dynamic_shift : ArithShift  BitShiftNumberSource=Input port  BitShiftDirection=Right
      settings: InputPortMap=u0,p1
  dynamic_shift1 : ArithShift  BitShiftNumberSource=Input port  BitShiftDirection=Right
      settings: InputPortMap=u0,p1
  xout : Outport  OutDataTypeStr=fixdt(1, 26, 15)  SampleTime=3.33333333333333e-08
  yout : Outport  Port=2  OutDataTypeStr=fixdt(1, 26, 15)  SampleTime=3.33333333333333e-08
  wires:
  MuxY/1 -> yout/1
  MuxX/1 -> xout/1
  YSub/1 -> MuxY/3
  YAdder/1 -> MuxY/1
  XAdder/1 -> MuxX/3
  XSubtractor/1 -> MuxX/1
  compare/1 -> MuxX/2, MuxY/2
  dynamic_shift/1 -> YAdder/2, YSub/2
  idx/1 -> dynamic_shift1/2, dynamic_shift/2
  dynamic_shift1/1 -> XSubtractor/2, XAdder/2
  yin/1 -> YAdder/1, dynamic_shift1/1, compare/1, YSub/1
  xin/1 -> dynamic_shift/1, XSubtractor/1, XAdder/1

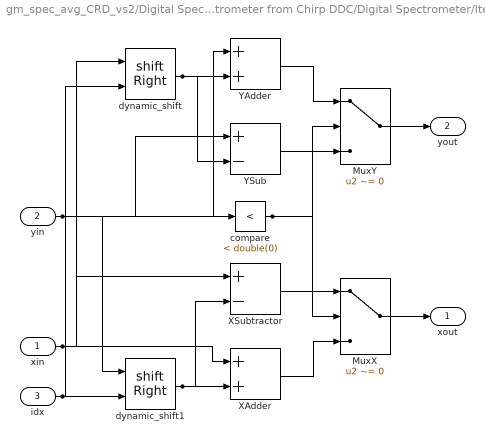
== system gm_spec_avg_CRD_vs2/Digital Spectrometer from Chirp DDC/Digital Spectrometer/Iteration1 ==
  xin : Inport  OutDataTypeStr=fixdt(1, 26, 15)  SampleTime=3.33333333333333e-08
  yin : Inport  Port=2  OutDataTypeStr=fixdt(1, 26, 15)  SampleTime=3.33333333333333e-08
  idx : Inport  Port=3  OutDataTypeStr=fixdt(0, 6, 0)  SampleTime=3.33333333333333e-08
  MuxX : Switch  Criteria=u2 ~= 0  Threshold="fi(0,0,1,0,\"hex\",\"0\")"  OutDataTypeStr=fixdt(1, 26, 15)  SampleTime=3.33333333333333e-08  SaturateOnIntegerOverflow=off  InputSameDT=off
  MuxY : Switch  Criteria=u2 ~= 0  Threshold="fi(0,0,1,0,\"hex\",\"0\")"  OutDataTypeStr=fixdt(1, 26, 15)  SampleTime=3.33333333333333e-08  SaturateOnIntegerOverflow=off  InputSameDT=off
  XAdder : Sum  OutDataTypeStr=fixdt(1, 26, 15)  SampleTime=3.33333333333333e-08
  XSubtractor : Sum  Inputs=+-  OutDataTypeStr=fixdt(1, 26, 15)  AccumDataTypeStr=fixdt(1, 26, 15)  SampleTime=3.33333333333333e-08
  YAdder : Sum  OutDataTypeStr=fixdt(1, 26, 15)  SampleTime=3.33333333333333e-08
  YSub : Sum  Inputs=+-  OutDataTypeStr=fixdt(1, 26, 15)  AccumDataTypeStr=fixdt(1, 26, 15)  SampleTime=3.33333333333333e-08
  compare : simulink/Logic and Bit Operations/Compare To Constant  relop=<  const=double(0)  OutDataTypeStr=boolean
  dynamic_shift : ArithShift  BitShiftNumberSource=Input port  BitShiftDirection=Right
      settings: InputPortMap=u0,p1
  dynamic_shift1 : ArithShift  BitShiftNumberSource=Input port  BitShiftDirection=Right
      settings: InputPortMap=u0,p1
  xout : Outport  OutDataTypeStr=fixdt(1, 26, 15)  SampleTime=3.33333333333333e-08
  yout : Outport  Port=2  OutDataTypeStr=fixdt(1, 26, 15)  SampleTime=3.33333333333333e-08
  wires:
  MuxX/1 -> xout/1
  MuxY/1 -> yout/1
  XAdder/1 -> MuxX/3
  XSubtractor/1 -> MuxX/1
  YAdder/1 -> MuxY/1
  compare/1 -> MuxY/2, MuxX/2
  idx/1 -> dynamic_shift1/2, dynamic_shift/2
  xin/1 -> dynamic_shift/1, XAdder/1, XSubtractor/1
  dynamic_shift1/1 -> XSubtractor/2, XAdder/2
  YSub/1 -> MuxY/3
  yin/1 -> dynamic_shift1/1, YAdder/1, YSub/1, compare/1
  dynamic_shift/1 -> YAdder/2, YSub/2

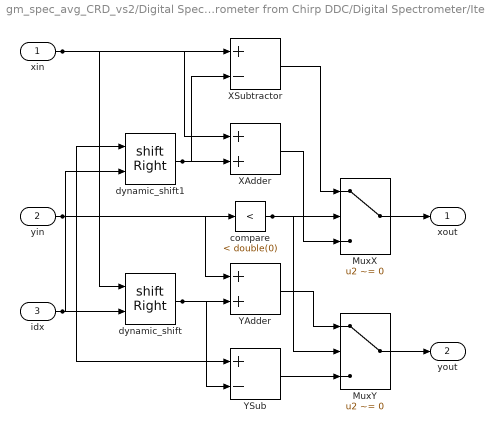
== system gm_spec_avg_CRD_vs2/Digital Spectrometer from Chirp DDC/Digital Spectrometer/Iteration10 ==
  xin : Inport  OutDataTypeStr=fixdt(1, 26, 15)  SampleTime=3.33333333333333e-08
  yin : Inport  Port=2  OutDataTypeStr=fixdt(1, 26, 15)  SampleTime=3.33333333333333e-08
  idx : Inport  Port=3  OutDataTypeStr=fixdt(0, 6, 0)  SampleTime=3.33333333333333e-08
  MuxX : Switch  Criteria=u2 ~= 0  Threshold="fi(0,0,1,0,\"hex\",\"0\")"  OutDataTypeStr=fixdt(1, 26, 15)  SampleTime=3.33333333333333e-08  SaturateOnIntegerOverflow=off  InputSameDT=off
  MuxY : Switch  Criteria=u2 ~= 0  Threshold="fi(0,0,1,0,\"hex\",\"0\")"  OutDataTypeStr=fixdt(1, 26, 15)  SampleTime=3.33333333333333e-08  SaturateOnIntegerOverflow=off  InputSameDT=off
  XAdder : Sum  OutDataTypeStr=fixdt(1, 26, 15)  SampleTime=3.33333333333333e-08
  XSubtractor : Sum  Inputs=+-  OutDataTypeStr=fixdt(1, 26, 15)  AccumDataTypeStr=fixdt(1, 26, 15)  SampleTime=3.33333333333333e-08
  YAdder : Sum  OutDataTypeStr=fixdt(1, 26, 15)  SampleTime=3.33333333333333e-08
  YSub : Sum  Inputs=+-  OutDataTypeStr=fixdt(1, 26, 15)  AccumDataTypeStr=fixdt(1, 26, 15)  SampleTime=3.33333333333333e-08
  compare : simulink/Logic and Bit Operations/Compare To Constant  relop=<  const=double(0)  OutDataTypeStr=boolean
  dynamic_shift : ArithShift  BitShiftNumberSource=Input port  BitShiftDirection=Right
      settings: InputPortMap=u0,p1
  dynamic_shift1 : ArithShift  BitShiftNumberSource=Input port  BitShiftDirection=Right
      settings: InputPortMap=u0,p1
  xout : Outport  OutDataTypeStr=fixdt(1, 26, 15)  SampleTime=3.33333333333333e-08
  yout : Outport  Port=2  OutDataTypeStr=fixdt(1, 26, 15)  SampleTime=3.33333333333333e-08
  wires:
  MuxX/1 -> xout/1
  YSub/1 -> MuxY/3
  YAdder/1 -> MuxY/1
  XAdder/1 -> MuxX/3
  XSubtractor/1 -> MuxX/1
  compare/1 -> MuxY/2, MuxX/2
  dynamic_shift1/1 -> XSubtractor/2, XAdder/2
  idx/1 -> dynamic_shift1/2, dynamic_shift/2
  yin/1 -> compare/1, dynamic_shift1/1, YAdder/1, YSub/1
  MuxY/1 -> yout/1
  dynamic_shift/1 -> YAdder/2, YSub/2
  xin/1 -> dynamic_shift/1, XSubtractor/1, XAdder/1

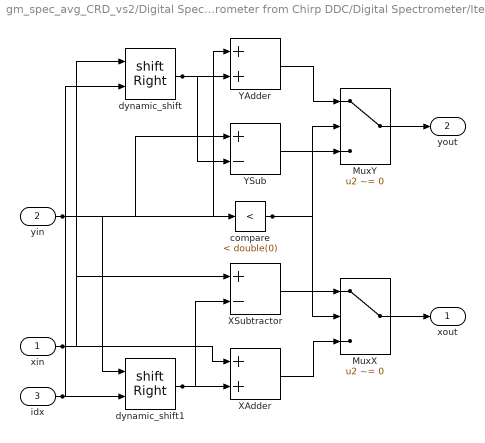
== system gm_spec_avg_CRD_vs2/Digital Spectrometer from Chirp DDC/Digital Spectrometer/Iteration11 ==
  xin : Inport  OutDataTypeStr=fixdt(1, 26, 15)  SampleTime=3.33333333333333e-08
  yin : Inport  Port=2  OutDataTypeStr=fixdt(1, 26, 15)  SampleTime=3.33333333333333e-08
  idx : Inport  Port=3  OutDataTypeStr=fixdt(0, 6, 0)  SampleTime=3.33333333333333e-08
  MuxX : Switch  Criteria=u2 ~= 0  Threshold="fi(0,0,1,0,\"hex\",\"0\")"  OutDataTypeStr=fixdt(1, 26, 15)  SampleTime=3.33333333333333e-08  SaturateOnIntegerOverflow=off  InputSameDT=off
  MuxY : Switch  Criteria=u2 ~= 0  Threshold="fi(0,0,1,0,\"hex\",\"0\")"  OutDataTypeStr=fixdt(1, 26, 15)  SampleTime=3.33333333333333e-08  SaturateOnIntegerOverflow=off  InputSameDT=off
  XAdder : Sum  OutDataTypeStr=fixdt(1, 26, 15)  SampleTime=3.33333333333333e-08
  XSubtractor : Sum  Inputs=+-  OutDataTypeStr=fixdt(1, 26, 15)  AccumDataTypeStr=fixdt(1, 26, 15)  SampleTime=3.33333333333333e-08
  YAdder : Sum  OutDataTypeStr=fixdt(1, 26, 15)  SampleTime=3.33333333333333e-08
  YSub : Sum  Inputs=+-  OutDataTypeStr=fixdt(1, 26, 15)  AccumDataTypeStr=fixdt(1, 26, 15)  SampleTime=3.33333333333333e-08
  compare : simulink/Logic and Bit Operations/Compare To Constant  relop=<  const=double(0)  OutDataTypeStr=boolean
  dynamic_shift : ArithShift  BitShiftNumberSource=Input port  BitShiftDirection=Right
      settings: InputPortMap=u0,p1
  dynamic_shift1 : ArithShift  BitShiftNumberSource=Input port  BitShiftDirection=Right
      settings: InputPortMap=u0,p1
  xout : Outport  OutDataTypeStr=fixdt(1, 26, 15)  SampleTime=3.33333333333333e-08
  yout : Outport  Port=2  OutDataTypeStr=fixdt(1, 26, 15)  SampleTime=3.33333333333333e-08
  wires:
  MuxY/1 -> yout/1
  XAdder/1 -> MuxX/3
  XSubtractor/1 -> MuxX/1
  YAdder/1 -> MuxY/1
  idx/1 -> dynamic_shift1/2, dynamic_shift/2
  MuxX/1 -> xout/1
  compare/1 -> MuxY/2, MuxX/2
  xin/1 -> dynamic_shift/1, XAdder/1, XSubtractor/1
  dynamic_shift1/1 -> XAdder/2, XSubtractor/2
  YSub/1 -> MuxY/3
  yin/1 -> compare/1, dynamic_shift1/1, YSub/1, YAdder/1
  dynamic_shift/1 -> YSub/2, YAdder/2

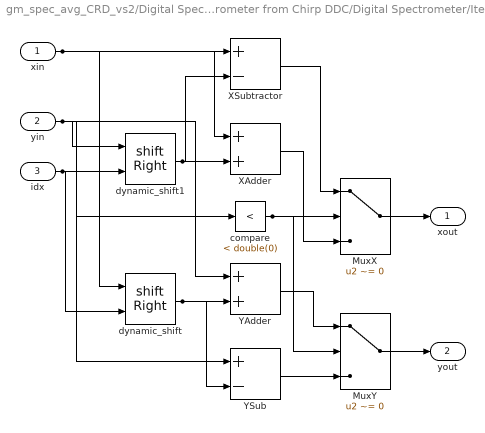
== system gm_spec_avg_CRD_vs2/Digital Spectrometer from Chirp DDC/Digital Spectrometer/Iteration12 ==
  xin : Inport  OutDataTypeStr=fixdt(1, 26, 15)  SampleTime=3.33333333333333e-08
  yin : Inport  Port=2  OutDataTypeStr=fixdt(1, 26, 15)  SampleTime=3.33333333333333e-08
  idx : Inport  Port=3  OutDataTypeStr=fixdt(0, 6, 0)  SampleTime=3.33333333333333e-08
  MuxX : Switch  Criteria=u2 ~= 0  Threshold="fi(0,0,1,0,\"hex\",\"0\")"  OutDataTypeStr=fixdt(1, 26, 15)  SampleTime=3.33333333333333e-08  SaturateOnIntegerOverflow=off  InputSameDT=off
  MuxY : Switch  Criteria=u2 ~= 0  Threshold="fi(0,0,1,0,\"hex\",\"0\")"  OutDataTypeStr=fixdt(1, 26, 15)  SampleTime=3.33333333333333e-08  SaturateOnIntegerOverflow=off  InputSameDT=off
  XAdder : Sum  OutDataTypeStr=fixdt(1, 26, 15)  SampleTime=3.33333333333333e-08
  XSubtractor : Sum  Inputs=+-  OutDataTypeStr=fixdt(1, 26, 15)  AccumDataTypeStr=fixdt(1, 26, 15)  SampleTime=3.33333333333333e-08
  YAdder : Sum  OutDataTypeStr=fixdt(1, 26, 15)  SampleTime=3.33333333333333e-08
  YSub : Sum  Inputs=+-  OutDataTypeStr=fixdt(1, 26, 15)  AccumDataTypeStr=fixdt(1, 26, 15)  SampleTime=3.33333333333333e-08
  compare : simulink/Logic and Bit Operations/Compare To Constant  relop=<  const=double(0)  OutDataTypeStr=boolean
  dynamic_shift : ArithShift  BitShiftNumberSource=Input port  BitShiftDirection=Right
      settings: InputPortMap=u0,p1
  dynamic_shift1 : ArithShift  BitShiftNumberSource=Input port  BitShiftDirection=Right
      settings: InputPortMap=u0,p1
  xout : Outport  OutDataTypeStr=fixdt(1, 26, 15)  SampleTime=3.33333333333333e-08
  yout : Outport  Port=2  OutDataTypeStr=fixdt(1, 26, 15)  SampleTime=3.33333333333333e-08
  wires:
  MuxY/1 -> yout/1
  MuxX/1 -> xout/1
  YSub/1 -> MuxY/3
  YAdder/1 -> MuxY/1
  XAdder/1 -> MuxX/3
  XSubtractor/1 -> MuxX/1
  compare/1 -> MuxX/2, MuxY/2
  dynamic_shift1/1 -> XSubtractor/2, XAdder/2
  idx/1 -> dynamic_shift/2, dynamic_shift1/2
  yin/1 -> YSub/1, dynamic_shift1/1, compare/1, YAdder/1
  dynamic_shift/1 -> YAdder/2, YSub/2
  xin/1 -> dynamic_shift/1, XSubtractor/1, XAdder/1

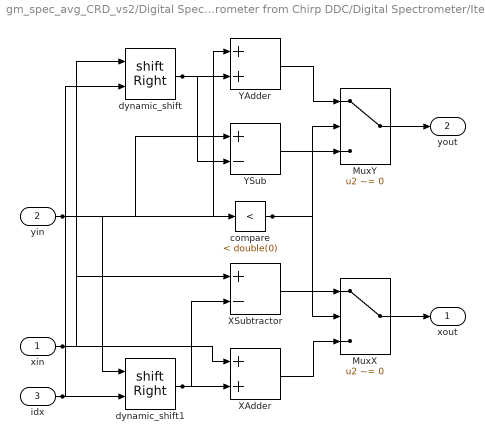
== system gm_spec_avg_CRD_vs2/Digital Spectrometer from Chirp DDC/Digital Spectrometer/Iteration13 ==
  xin : Inport  OutDataTypeStr=fixdt(1, 26, 15)  SampleTime=3.33333333333333e-08
  yin : Inport  Port=2  OutDataTypeStr=fixdt(1, 26, 15)  SampleTime=3.33333333333333e-08
  idx : Inport  Port=3  OutDataTypeStr=fixdt(0, 6, 0)  SampleTime=3.33333333333333e-08
  MuxX : Switch  Criteria=u2 ~= 0  Threshold="fi(0,0,1,0,\"hex\",\"0\")"  OutDataTypeStr=fixdt(1, 26, 15)  SampleTime=3.33333333333333e-08  SaturateOnIntegerOverflow=off  InputSameDT=off
  MuxY : Switch  Criteria=u2 ~= 0  Threshold="fi(0,0,1,0,\"hex\",\"0\")"  OutDataTypeStr=fixdt(1, 26, 15)  SampleTime=3.33333333333333e-08  SaturateOnIntegerOverflow=off  InputSameDT=off
  XAdder : Sum  OutDataTypeStr=fixdt(1, 26, 15)  SampleTime=3.33333333333333e-08
  XSubtractor : Sum  Inputs=+-  OutDataTypeStr=fixdt(1, 26, 15)  AccumDataTypeStr=fixdt(1, 26, 15)  SampleTime=3.33333333333333e-08
  YAdder : Sum  OutDataTypeStr=fixdt(1, 26, 15)  SampleTime=3.33333333333333e-08
  YSub : Sum  Inputs=+-  OutDataTypeStr=fixdt(1, 26, 15)  AccumDataTypeStr=fixdt(1, 26, 15)  SampleTime=3.33333333333333e-08
  compare : simulink/Logic and Bit Operations/Compare To Constant  relop=<  const=double(0)  OutDataTypeStr=boolean
  dynamic_shift : ArithShift  BitShiftNumberSource=Input port  BitShiftDirection=Right
      settings: InputPortMap=u0,p1
  dynamic_shift1 : ArithShift  BitShiftNumberSource=Input port  BitShiftDirection=Right
      settings: InputPortMap=u0,p1
  xout : Outport  OutDataTypeStr=fixdt(1, 26, 15)  SampleTime=3.33333333333333e-08
  yout : Outport  Port=2  OutDataTypeStr=fixdt(1, 26, 15)  SampleTime=3.33333333333333e-08
  wires:
  XAdder/1 -> MuxX/3
  XSubtractor/1 -> MuxX/1
  YAdder/1 -> MuxY/1
  dynamic_shift1/1 -> XAdder/2, XSubtractor/2
  YSub/1 -> MuxY/3
  idx/1 -> dynamic_shift1/2, dynamic_shift/2
  MuxX/1 -> xout/1
  compare/1 -> MuxY/2, MuxX/2
  xin/1 -> dynamic_shift/1, XAdder/1, XSubtractor/1
  MuxY/1 -> yout/1
  yin/1 -> dynamic_shift1/1, compare/1, YSub/1, YAdder/1
  dynamic_shift/1 -> YAdder/2, YSub/2

== system gm_spec_avg_CRD_vs2/Digital Spectrometer from Chirp DDC/Digital Spectrometer/Iteration14 ==
  xin : Inport  OutDataTypeStr=fixdt(1, 26, 15)  SampleTime=3.33333333333333e-08
  yin : Inport  Port=2  OutDataTypeStr=fixdt(1, 26, 15)  SampleTime=3.33333333333333e-08
  idx : Inport  Port=3  OutDataTypeStr=fixdt(0, 6, 0)  SampleTime=3.33333333333333e-08
  MuxX : Switch  Criteria=u2 ~= 0  Threshold="fi(0,0,1,0,\"hex\",\"0\")"  OutDataTypeStr=fixdt(1, 26, 15)  SampleTime=3.33333333333333e-08  SaturateOnIntegerOverflow=off  InputSameDT=off
  MuxY : Switch  Criteria=u2 ~= 0  Threshold="fi(0,0,1,0,\"hex\",\"0\")"  OutDataTypeStr=fixdt(1, 26, 15)  SampleTime=3.33333333333333e-08  SaturateOnIntegerOverflow=off  InputSameDT=off
  XAdder : Sum  OutDataTypeStr=fixdt(1, 26, 15)  SampleTime=3.33333333333333e-08
  XSubtractor : Sum  Inputs=+-  OutDataTypeStr=fixdt(1, 26, 15)  AccumDataTypeStr=fixdt(1, 26, 15)  SampleTime=3.33333333333333e-08
  YAdder : Sum  OutDataTypeStr=fixdt(1, 26, 15)  SampleTime=3.33333333333333e-08
  YSub : Sum  Inputs=+-  OutDataTypeStr=fixdt(1, 26, 15)  AccumDataTypeStr=fixdt(1, 26, 15)  SampleTime=3.33333333333333e-08
  compare : simulink/Logic and Bit Operations/Compare To Constant  relop=<  const=double(0)  OutDataTypeStr=boolean
  dynamic_shift : ArithShift  BitShiftNumberSource=Input port  BitShiftDirection=Right
      settings: InputPortMap=u0,p1
  dynamic_shift1 : ArithShift  BitShiftNumberSource=Input port  BitShiftDirection=Right
      settings: InputPortMap=u0,p1
  xout : Outport  OutDataTypeStr=fixdt(1, 26, 15)  SampleTime=3.33333333333333e-08
  yout : Outport  Port=2  OutDataTypeStr=fixdt(1, 26, 15)  SampleTime=3.33333333333333e-08
  wires:
  MuxY/1 -> yout/1
  MuxX/1 -> xout/1
  YSub/1 -> MuxY/3
  YAdder/1 -> MuxY/1
  XAdder/1 -> MuxX/3
  XSubtractor/1 -> MuxX/1
  compare/1 -> MuxX/2, MuxY/2
  dynamic_shift1/1 -> XSubtractor/2, XAdder/2
  idx/1 -> dynamic_shift/2, dynamic_shift1/2
  yin/1 -> YAdder/1, dynamic_shift1/1, compare/1, YSub/1
  dynamic_shift/1 -> YAdder/2, YSub/2
  xin/1 -> dynamic_shift/1, XSubtractor/1, XAdder/1

== system gm_spec_avg_CRD_vs2/Digital Spectrometer from Chirp DDC/Digital Spectrometer/Iteration15 ==
  xin : Inport  OutDataTypeStr=fixdt(1, 26, 15)  SampleTime=3.33333333333333e-08
  yin : Inport  Port=2  OutDataTypeStr=fixdt(1, 26, 15)  SampleTime=3.33333333333333e-08
  idx : Inport  Port=3  OutDataTypeStr=fixdt(0, 6, 0)  SampleTime=3.33333333333333e-08
  MuxX : Switch  Criteria=u2 ~= 0  Threshold="fi(0,0,1,0,\"hex\",\"0\")"  OutDataTypeStr=fixdt(1, 26, 15)  SampleTime=3.33333333333333e-08  SaturateOnIntegerOverflow=off  InputSameDT=off
  MuxY : Switch  Criteria=u2 ~= 0  Threshold="fi(0,0,1,0,\"hex\",\"0\")"  OutDataTypeStr=fixdt(1, 26, 15)  SampleTime=3.33333333333333e-08  SaturateOnIntegerOverflow=off  InputSameDT=off
  XAdder : Sum  OutDataTypeStr=fixdt(1, 26, 15)  SampleTime=3.33333333333333e-08
  XSubtractor : Sum  Inputs=+-  OutDataTypeStr=fixdt(1, 26, 15)  AccumDataTypeStr=fixdt(1, 26, 15)  SampleTime=3.33333333333333e-08
  YAdder : Sum  OutDataTypeStr=fixdt(1, 26, 15)  SampleTime=3.33333333333333e-08
  YSub : Sum  Inputs=+-  OutDataTypeStr=fixdt(1, 26, 15)  AccumDataTypeStr=fixdt(1, 26, 15)  SampleTime=3.33333333333333e-08
  compare : simulink/Logic and Bit Operations/Compare To Constant  relop=<  const=double(0)  OutDataTypeStr=boolean
  dynamic_shift : ArithShift  BitShiftNumberSource=Input port  BitShiftDirection=Right
      settings: InputPortMap=u0,p1
  dynamic_shift1 : ArithShift  BitShiftNumberSource=Input port  BitShiftDirection=Right
      settings: InputPortMap=u0,p1
  xout : Outport  OutDataTypeStr=fixdt(1, 26, 15)  SampleTime=3.33333333333333e-08
  yout : Outport  Port=2  OutDataTypeStr=fixdt(1, 26, 15)  SampleTime=3.33333333333333e-08
  wires:
  MuxY/1 -> yout/1
  XAdder/1 -> MuxX/3
  XSubtractor/1 -> MuxX/1
  YAdder/1 -> MuxY/1
  idx/1 -> dynamic_shift1/2, dynamic_shift/2
  MuxX/1 -> xout/1
  compare/1 -> MuxY/2, MuxX/2
  xin/1 -> dynamic_shift/1, XAdder/1, XSubtractor/1
  dynamic_shift1/1 -> XAdder/2, XSubtractor/2
  YSub/1 -> MuxY/3
  yin/1 -> dynamic_shift1/1, YSub/1, compare/1, YAdder/1
  dynamic_shift/1 -> YSub/2, YAdder/2

== system gm_spec_avg_CRD_vs2/Digital Spectrometer from Chirp DDC/Digital Spectrometer/Iteration16 ==
  xin : Inport  OutDataTypeStr=fixdt(1, 26, 15)  SampleTime=3.33333333333333e-08
  yin : Inport  Port=2  OutDataTypeStr=fixdt(1, 26, 15)  SampleTime=3.33333333333333e-08
  idx : Inport  Port=3  OutDataTypeStr=fixdt(0, 6, 0)  SampleTime=3.33333333333333e-08
  MuxX : Switch  Criteria=u2 ~= 0  Threshold="fi(0,0,1,0,\"hex\",\"0\")"  OutDataTypeStr=fixdt(1, 26, 15)  SampleTime=3.33333333333333e-08  SaturateOnIntegerOverflow=off  InputSameDT=off
  MuxY : Switch  Criteria=u2 ~= 0  Threshold="fi(0,0,1,0,\"hex\",\"0\")"  OutDataTypeStr=fixdt(1, 26, 15)  SampleTime=3.33333333333333e-08  SaturateOnIntegerOverflow=off  InputSameDT=off
  XAdder : Sum  OutDataTypeStr=fixdt(1, 26, 15)  SampleTime=3.33333333333333e-08
  XSubtractor : Sum  Inputs=+-  OutDataTypeStr=fixdt(1, 26, 15)  AccumDataTypeStr=fixdt(1, 26, 15)  SampleTime=3.33333333333333e-08
  YAdder : Sum  OutDataTypeStr=fixdt(1, 26, 15)  SampleTime=3.33333333333333e-08
  YSub : Sum  Inputs=+-  OutDataTypeStr=fixdt(1, 26, 15)  AccumDataTypeStr=fixdt(1, 26, 15)  SampleTime=3.33333333333333e-08
  compare : simulink/Logic and Bit Operations/Compare To Constant  relop=<  const=double(0)  OutDataTypeStr=boolean
  dynamic_shift : ArithShift  BitShiftNumberSource=Input port  BitShiftDirection=Right
      settings: InputPortMap=u0,p1
  dynamic_shift1 : ArithShift  BitShiftNumberSource=Input port  BitShiftDirection=Right
      settings: InputPortMap=u0,p1
  xout : Outport  OutDataTypeStr=fixdt(1, 26, 15)  SampleTime=3.33333333333333e-08
  yout : Outport  Port=2  OutDataTypeStr=fixdt(1, 26, 15)  SampleTime=3.33333333333333e-08
  wires:
  MuxY/1 -> yout/1
  MuxX/1 -> xout/1
  YSub/1 -> MuxY/3
  YAdder/1 -> MuxY/1
  XAdder/1 -> MuxX/3
  XSubtractor/1 -> MuxX/1
  compare/1 -> MuxX/2, MuxY/2
  dynamic_shift1/1 -> XSubtractor/2, XAdder/2
  idx/1 -> dynamic_shift/2, dynamic_shift1/2
  yin/1 -> dynamic_shift1/1, compare/1, YAdder/1, YSub/1
  dynamic_shift/1 -> YAdder/2, YSub/2
  xin/1 -> XAdder/1, dynamic_shift/1, XSubtractor/1
